simulink model "rangeSensorStart"  (R2018a)
settings: Solver=FixedStepDiscrete  StartTime=0.0  StopTime=10.0  RelTol=1e-3
PreLoadFcn:
  | tFilter = 0.01;
  | tFusion = 0.05;
  | 
  | sensData = dlmread('rangeSensorData.txt');
settings Model: Creator=scastro  LastModifiedBy=scastro
settings DataIOCC: ExternalInput=sensData  LoadExternalInput=on
settings OptimizationCC: DefaultParameterBehavior=Inlined  EnhancedBackFolding=on  PassReuseOutputArgsAs=Individual arguments  OptimizeBlockOrder=speed  DifferentSizesBufferReuse=on  OptimizationCustomize=off
settings DebuggingCC: ParameterTunabilityLossMsg=error  LibraryContextMissingDiagnostic=warning
settings SFSimCC: SimUseLocalCustomCode=on  MATLABDynamicMemAlloc=off
settings RTWCC: SystemTargetFile=ert.tlc  TemplateMakefile=ert_default_tmf  GenerateReport=on  RTWUseLocalCustomCode=on  IncludeHyperlinkInReport=on  LaunchReport=on  GenerateTraceInfo=on  GenerateTraceReport=on  GenerateTraceReportSl=on  GenerateTraceReportSf=on  GenerateTraceReportEml=on
settings CodeAppCC: ForceParamTrailComments=on  IgnoreCustomStorageClasses=off  OperatorAnnotations=on  SimulinkDataObjDesc=on  SFDataObjDesc=on  InsertBlockDesc=on
settings ERTTargetCC: TargetLangStandard=C99 (ISO)  GenerateSampleERTMain=on  InlinedParameterPlacement=NonHierarchical  ERTCustomFileTemplate=example_file_process.tlc

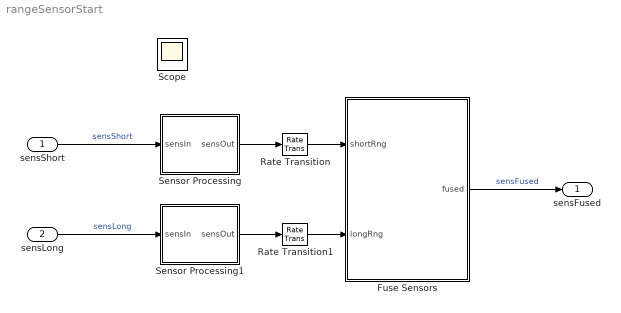
== system rangeSensorStart ==
  sensShort : Inport
  sensLong : Inport  Port=2
  Fuse Sensors : Stateflow chart  TreatAsAtomicUnit=on  SystemSampleTime=tFusion
  Rate Transition : RateTransition
  Rate Transition1 : RateTransition
  Sensor Processing : Subsystem
  Sensor Processing1 : Subsystem
  sensFused : Outport
  Scope : Scope
  wires:
  Sensor Processing/1(sensOut) -> Rate Transition/1
  sensShort/1 -> Sensor Processing/1(sensIn)  "sensShort"
  Sensor Processing1/1(sensOut) -> Rate Transition1/1
  sensLong/1 -> Sensor Processing1/1(sensIn)  "sensLong"
  Fuse Sensors/1(fused) -> sensFused/1  "sensFused"
  Rate Transition/1 -> Fuse Sensors/1(shortRng)
  Rate Transition1/1 -> Fuse Sensors/2(longRng)

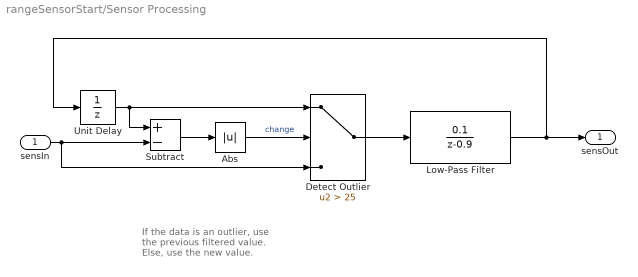
== system rangeSensorStart/Sensor Processing ==
  note: If the data is an outlier, use the previous filtered value.
      | Else, use the new value.
  sensIn : Inport
  Abs : Abs
  Detect Outlier : Switch  Criteria=u2 > Threshold  Threshold=25
  Low-Pass Filter : DiscreteTransferFcn  Numerator=[0.1]  Denominator=[1 -0.9]  SampleTime=tFilter
  Subtract : Sum  Inputs=+-
  Unit Delay : UnitDelay  SampleTime=-1
  sensOut : Outport
  wires:
  sensIn/1 -> Subtract/2, Detect Outlier/3
  Detect Outlier/1 -> Low-Pass Filter/1
  Low-Pass Filter/1 -> sensOut/1, Unit Delay/1
  Unit Delay/1 -> Subtract/1, Detect Outlier/1
  Abs/1 -> Detect Outlier/2  "change"
  Subtract/1 -> Abs/1

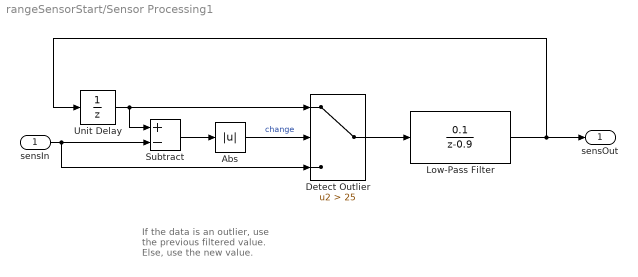
== system rangeSensorStart/Sensor Processing1 ==
  note: If the data is an outlier, use the previous filtered value.
      | Else, use the new value.
  sensIn : Inport
  Abs : Abs
  Detect Outlier : Switch  Criteria=u2 > Threshold  Threshold=25
  Low-Pass Filter : DiscreteTransferFcn  Numerator=[0.1]  Denominator=[1 -0.9]  SampleTime=tFilter
  Subtract : Sum  Inputs=+-
  Unit Delay : UnitDelay  SampleTime=-1
  sensOut : Outport
  wires:
  Subtract/1 -> Abs/1
  Abs/1 -> Detect Outlier/2  "change"
  Unit Delay/1 -> Detect Outlier/1, Subtract/1
  Low-Pass Filter/1 -> Unit Delay/1, sensOut/1
  Detect Outlier/1 -> Low-Pass Filter/1
  sensIn/1 -> Detect Outlier/3, Subtract/2

== stateflow chart rangeSensorStart/Fuse Sensors ==
  state AverageReadings
    en,du:
    fused = 0.5*(shortRng + longRng);
  state ShortRange
    en,du:
    fused = shortRng;
  state LongRange
    en,du:
    fused = longRng;
  (default) -> AverageReadings
  AverageReadings -> LongRange [order 2] : [fused > 80]
  AverageReadings -> ShortRange [order 1] : [fused < 40]
  LongRange -> AverageReadings : [fused <= 80]
  ShortRange -> AverageReadings : [fused >= 40]
  data: shortRng input; longRng input; fused output
